simulink model "bbcSimPID"  (R2024b)
settings: Solver=FixedStepDiscrete  StartTime=0.0  StopTime=0.15  FixedStep=5e-6  RelTol=1e-3
model workspace (MAT data in the model file):
  vIn = 48
libraries: spsSeriesRLCBranchLib x3, spsVoltageMeasurementLib x2, spsDiodeLib x1, spsMosfetLib x1, spsDCVoltageSourceLib x1, spspowerguiLib x1, spsPWMGeneratorDCDCLib x1
settings Model: Creator=mattf  LastModifiedBy=nicholas

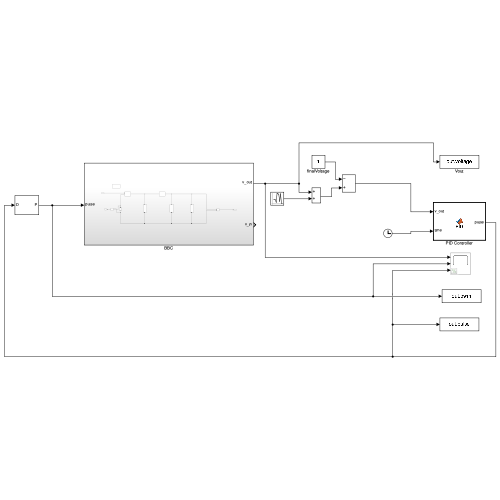
[thumbnail: Simulink's stored preview of the top-level diagram]
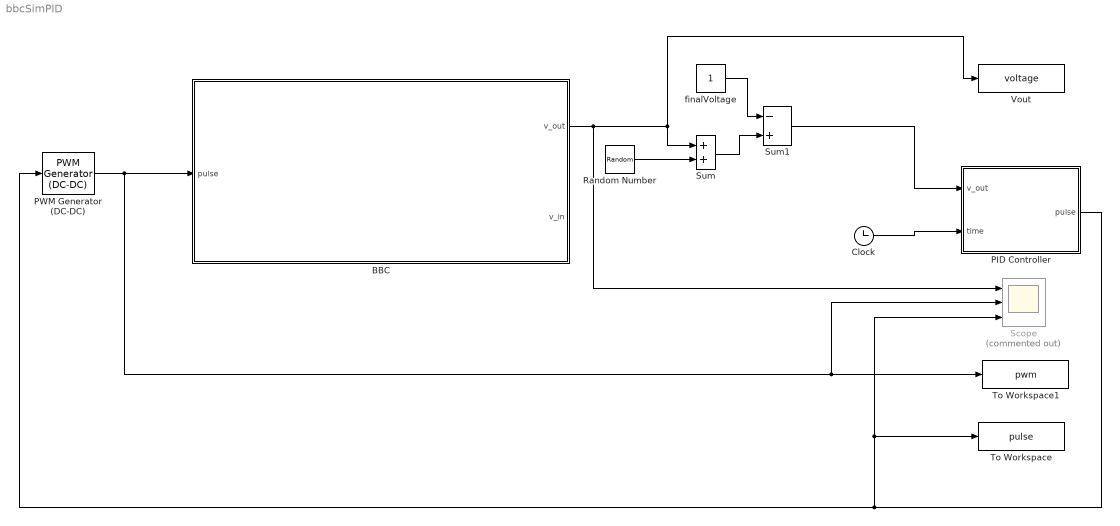
== system bbcSimPID ==
  BBC : Subsystem
  Clock : Clock
  PID Controller : MATLAB Function  TreatAsAtomicUnit=on
  PWM Generator (DC-DC) : spsPWMGeneratorDCDCLib/PWM Generator (DC-DC)  Fsw=7.8e3  Ts=5e-6
  Random Number : RandomNumber  Variance=0  SampleTime=5e-6
  Scope : Scope  Commented=on  NumInputPorts=3
  Sum : Sum
  Sum1 : Sum  Inputs=-+
  To Workspace : ToWorkspace  VariableName=pulse  SampleTime=-1
  To Workspace1 : ToWorkspace  VariableName=pwm  SampleTime=-1
  Vout : ToWorkspace  VariableName=voltage  SampleTime=-1
  finalVoltage : Constant
  wires:
  Clock/1 -> PID Controller/2(time)
  PWM Generator (DC-DC)/1 -> Scope/2, To Workspace1/1, BBC/1(pulse)
  PID Controller/1(pulse) -> PWM Generator (DC-DC)/1, Scope/3, To Workspace/1
  Random Number/1 -> Sum/2
  BBC/1(v_out) -> Vout/1, Sum/1, Scope/1
  finalVoltage/1 -> Sum1/1
  Sum/1 -> Sum1/2
  Sum1/1 -> PID Controller/1(v_out)

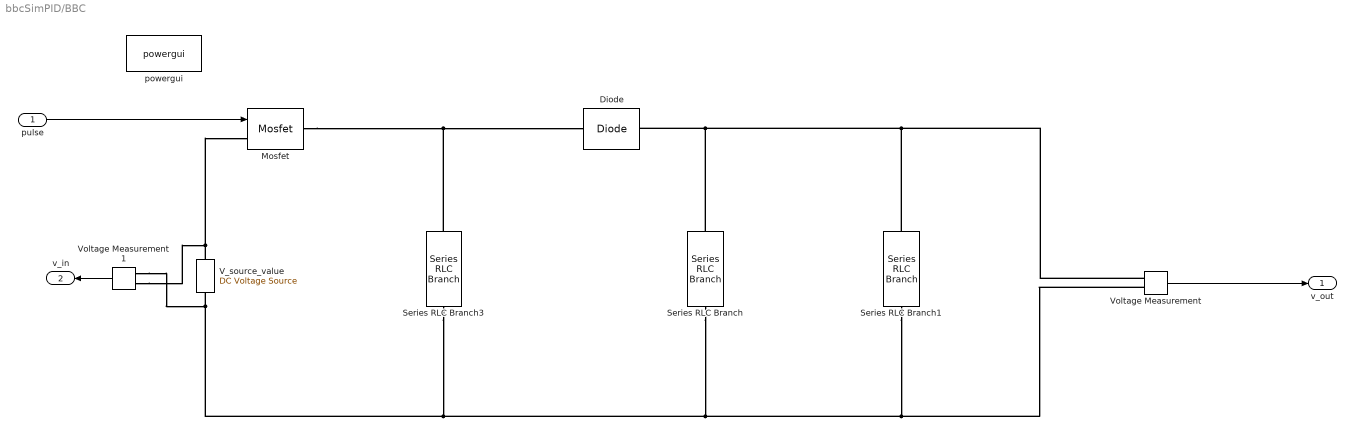
== system bbcSimPID/BBC ==
  pulse : Inport
  Diode : spsDiodeLib/Diode  Ron=0.001  Lon=0  Vf=0.8  IC=0  UseSnubber=0  Rs=500  Cs=250e-9  Measurements=off
  Mosfet : spsMosfetLib/Mosfet  Ron=0.1  Lon=0  Rd=0.01  Vfd=0  IC=0  Rs=1e5  Cs=inf  Measurements=off
  Series RLC Branch : spsSeriesRLCBranchLib/Series RLC Branch  LConnTagsString=__new0  RConnTagsString=__new0  BranchType=C  Resistance=1  Inductance=1e-3  SetiL0=off  InitialCurrent=0  Capacitance=8200e-6  Setx0=off  InitialVoltage=0  Measurements=None
  Series RLC Branch1 : spsSeriesRLCBranchLib/Series RLC Branch  LConnTagsString=__new0  RConnTagsString=__new0  BranchType=R  Resistance=5.1  Inductance=1e-3  SetiL0=off  InitialCurrent=0  Capacitance=1e-6  Setx0=off  InitialVoltage=0  Measurements=None
  Series RLC Branch3 : spsSeriesRLCBranchLib/Series RLC Branch  LConnTagsString=__new0  RConnTagsString=__new0  BranchType=L  Resistance=1  Inductance=220e-6  SetiL0=off  InitialCurrent=0  Capacitance=1e-6  Setx0=off  InitialVoltage=0  Measurements=None
  V_source_value : spsDCVoltageSourceLib/DC Voltage Source  Amplitude=48  Measurements=Voltage
  Voltage Measurement : spsVoltageMeasurementLib/Voltage Measurement  PhasorSimulation=off  OutputType=Complex  PSBequivalent=0
  Voltage Measurement1 : spsVoltageMeasurementLib/Voltage Measurement  PhasorSimulation=off  OutputType=Complex  PSBequivalent=0
  powergui : spspowerguiLib/powergui  Priority=1  SimulationMode=Discrete  SampleTime=5e-6  frequency=60  Iterations=50  frequencyindice=0  Pbase=100e6  ErrMax=1e-4  UnitsV=kV  UnitsW=MW  buscounter=0  FunctionMessages=off  echomessages=off  EnableUseOfTLC=off  CurrentSourceSwitches=off  DisableSnubberDevices=off  DisableRonSwitches=off  DisableVfSwitches=off  DisplayEquations=off  AutomaticDiscreteSolvers=off  SolverType=Tustin/Backward Euler (TBE)  Interpol=off  ExternalGateDelay=off  methode=off  Ts=100  x0status=blocks  SPID=on  SwTol=0  HookPort=off  NonlinearTolerance=1e-4  nMaxIteration=100  ContinueOnMaxIteration=off  RestoreLinks=warning  ResistiveCurrentMeasurement=off  Frange=[0:2:500]  Ylog=off  Xlog=on  ShowGrid=off  save=off  variable=ZData  structure=0  ZoomFFT=off  StartTime=0.0  cycles=1  DisplayStyle=1  fundamental=60  FreqAxis=off  MaxFrequency=1000  frequencyindicesteady=1  RmsSteady=1  display=off
  v_out : Outport
  v_in : Outport  Port=2
  wires:
  pulse/1 -> Mosfet/1
  Voltage Measurement/1 -> v_out/1
  Voltage Measurement1/1 -> v_in/1
  connections:
  V_source_value/RConn1 -- Voltage Measurement1/LConn1 -- Mosfet/LConn1
  Mosfet/RConn1 -- Series RLC Branch3/LConn1 -- Diode/RConn1
  Voltage Measurement/LConn2 -- Series RLC Branch1/RConn1 -- Series RLC Branch/RConn1 -- Series RLC Branch3/RConn1 -- Voltage Measurement1/LConn2 -- V_source_value/LConn1
  Voltage Measurement/LConn1 -- Series RLC Branch1/LConn1 -- Series RLC Branch/LConn1 -- Diode/LConn1

== matlab function bbcSimPID/PID Controller ==
  settings: updateMethod=DISCRETE
  data: v_out input; pulse output; time input
function pulse = PID(v_out, time)

    % call extrinsic python function
    coder.extrinsic('py.PIDControllerBBC.controller_call');

    % Call Python function and return result
    pulse = coder.nullcopy(zeros(1,1)); % no clue why, but this is need.
    pulse = double(py.PIDControllerBBC.controller_call(v_out, time));
    end
